simulink model "blood_sugar"  (R2022b)
settings: Solver=VariableStepAuto  StartTime=0.0  StopTime=200  RelTol=1e-3
undefined symbols (not defined in the file): ai, beta, lambda
settings Model: Creator=86133  LastModifiedBy=86133

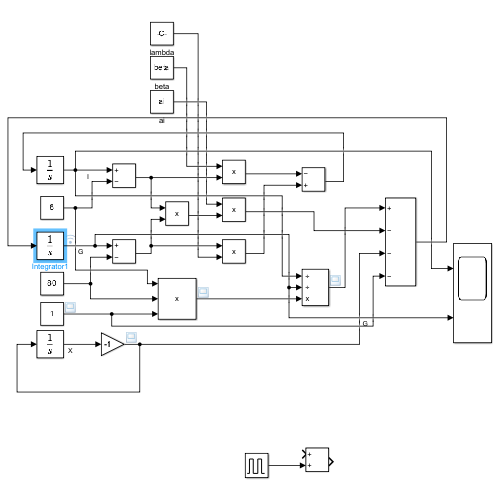
[thumbnail: Simulink's stored preview of the top-level diagram]
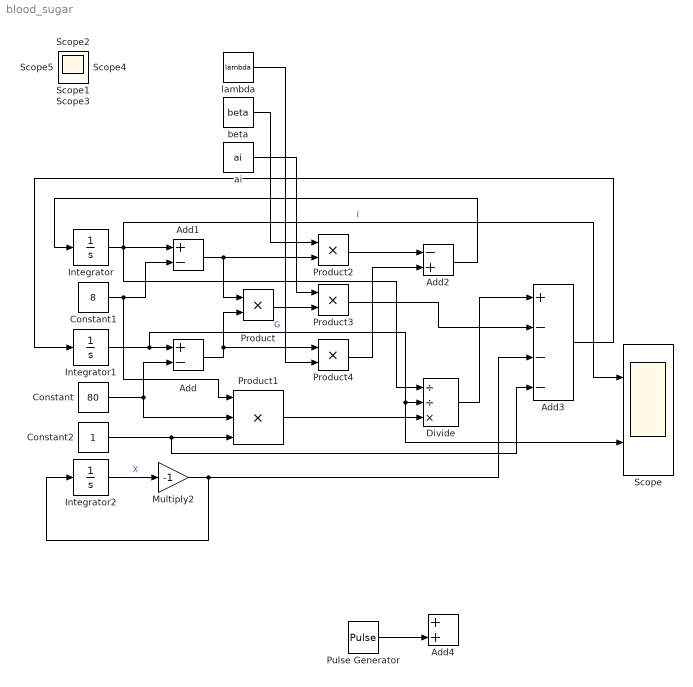
== system blood_sugar ==
  Add : Sum  Inputs=+-
  Add1 : Sum  Inputs=+-
  Add2 : Sum  Inputs=-+
  Add3 : Sum  Inputs=+---
  Add4 : Sum
  Constant : Constant  Value=80
  Constant1 : Constant  Value=8
  Constant2 : Constant
  Divide : Product  Inputs=//*
  Integrator : Integrator  InitialCondition=8
  Integrator1 : Integrator  InitialCondition=80
  Integrator2 : Integrator  InitialCondition=300
  Multiply2 : Gain  Gain=-1
  Product{,2..4} (4 alike) : Product
  Product1 : Product  Inputs=3
  Pulse Generator : DiscretePulseGenerator  PulseType=Time based  Amplitude=10000  Period=6  PulseWidth=0.15
  Scope : Scope  NumInputPorts=2
  ai : Constant  Value=ai
  beta : Constant  Value=beta
  lambda : Constant  Value=lambda
  Scope{1..5} (5 alike) : Scope
  wires:
  Integrator1/1 -> Scope/2, Divide/2, Add/1  "G"
  Constant/1 -> Product1/2, Add/2
  Add/1 -> Product4/1, Product/2
  Integrator/1 -> Scope/1, Divide/1, Add1/1  "I"
  Constant1/1 -> Product1/1, Add1/2
  Add1/1 -> Product2/2, Product/1
  Product2/1 -> Add2/1
  Product4/1 -> Add2/2
  Add2/1 -> Integrator/1
  Integrator2/1 -> Multiply2/1  "X"
  Product/1 -> Product3/2
  Constant2/1 -> Add3/4, Product1/3
  Product1/1 -> Divide/3
  Divide/1 -> Add3/1
  Add3/1 -> Integrator1/1
  Multiply2/1 -> Integrator2/1, Add3/3
  Pulse Generator/1 -> Add4/2
  Product3/1 -> Add3/2
  beta/1 -> Product2/1
  ai/1 -> Product3/1
  lambda/1 -> Product4/2
